simulink model "Implementation"  (Simulink 7.8)
settings: Solver=FixedStepDiscrete  StartTime=0.0  StopTime=inf  FixedStep=T  RelTol=1e-3
values from neighbouring files (symbols this model uses):
  A = [zeros(2,2),    eye(2,2) ... (first row only)    [StateFeedback_Controller_Observer_Design.m]    (also in equilibriumpositon_2_realsim.mat = [0 0 1.86000056553 -118.859256664 0 0 -4.86792536172 -131.56)
  B = [zeros(2,2) ... (first row only)    [StateFeedback_Controller_Observer_Design.m]    (also in equilibriumpositon_2_realsim.mat = [0 0 0.0946459156765 0.178753935587])
  C = [h*q2dot   h*(q1dot+q2dot) ... (first row only)    [NonLinModel.m]    (also in StateFeedback_Controller_Observer_Design.m = [1 0 0 0; equilibriumpositon_2_realsim.mat = [1  0  0  0; 0  1  0  0])
  K = place(A,B,p)    [StateFeedback_Controller_Observer_Design.m]    (also in equilibriumpositon_2_realsim.mat = [3103.64468197 1789.25362632 433.04949119 3.48374472995])
  L = transpose(place(A', C',po))    [StateFeedback_Controller_Observer_Design.m]    (also in equilibriumpositon_2_realsim.mat = [220.529108681  -24.0242041595; -32.2456951439  226.07999002)
  NewPanto = 1    [StateFeedback_Controller_Observer_Design.m]    (also in equilibriumpositon_2_realsim.mat = 0)
  q1 = x(1)    [NonLinModel.m]    (also in StateFeedback_Controller_Observer_Design.m = 1.57079632679; equilibriumpositon_2_realsim.mat = 1.57079632679)
  q2 = x(2)    [NonLinModel.m]    (also in StateFeedback_Controller_Observer_Design.m = 0; equilibriumpositon_2_realsim.mat = 3.14159265359)
  T = .001    (= 0.001)    [StateFeedback_Controller_Observer_Design.m]    (also in equilibriumpositon_2_realsim.mat)
undefined symbols (not defined in the file or in its folder): DiscIntNeverNeededParam, HIL, qc_get_step_size
libraries: quarc_library x5
settings Model: Creator=jafarm2  LastModifiedBy=jafarm2  SimulationMode=external  ExtModeTrigDuration=500000
settings SolverCC: PositivePriorityOrder=on
settings RTWCC: SystemTargetFile=quarc_win64.tlc  TemplateMakefile=quarc_default_tmf  Description=QUARC Win64 Target  ProcessScript=quarc_win64_make_rtw_hook
settings STFCustomTargetCC: TargetPreCompLibLocation=C:\PROGRA~3\QUARC\lib\2011b\win64\release  SystemTargetFile=quarc_win64.tlc
settings GRTTargetCC: TargetPreCompLibLocation=C:\PROGRA~3\QUARC\lib\2011b\win64\release  ParMdlRefBuildCompliant=off  CompOptLevelCompliant=off  ConcurrentExecutionCompliant=off  MatFileLogging=off  ExtMode=on  ExtModeMexFile=quarc_comm

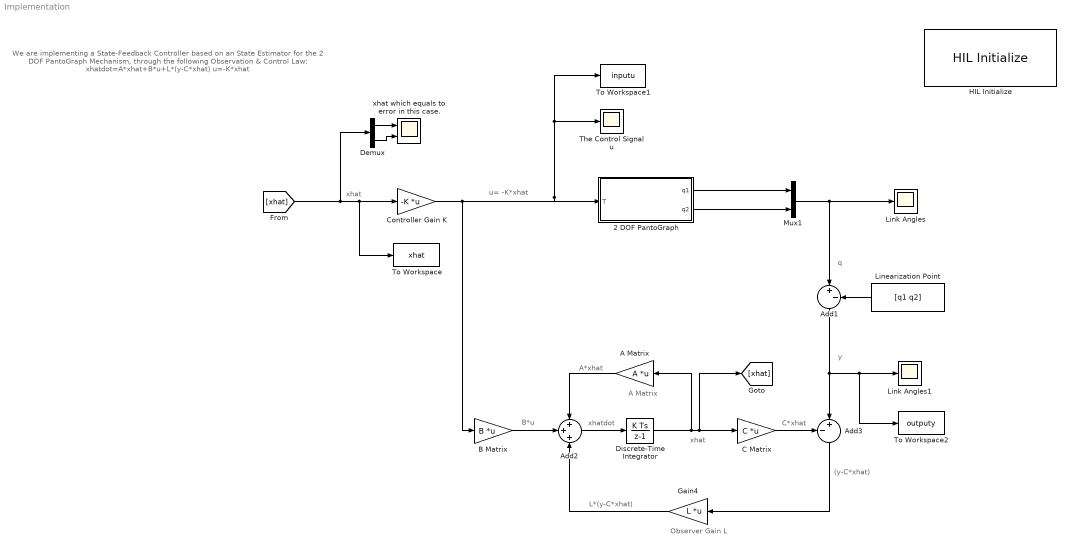
== system Implementation ==
  note: q
  note: y
  note: B*u
  note: A Matrix
  note: A*xhat
  note: xhat
  note: C*xhat
  note: (y-C*xhat)
  note: L*(y-C*xhat)
  note: Observer Gain L
  note: u= -K*xhat
  note: xhat
  note: xhatdot
  note: We are implementing a State-Feedback Controller based on an State Estimator for the 2 DOF PantoGraph Mechanism,
      | through the following Observation & Control Law:
      | xhatdot=A*xhat+B*u+L*(y-C*xhat)
      | u=-K*xhat
  2 DOF PantoGraph : Subsystem
  A Matrix : Gain  Gain=A  Multiplication=Matrix(K*u)
  Add1 : Sum  Inputs=|+-
  Add2 : Sum  Inputs=+++
  Add3 : Sum  Inputs=-+|
  B Matrix : Gain  Gain=B  Multiplication=Matrix(K*u)
  C Matrix : Gain  Gain=C  Multiplication=Matrix(K*u)
  Controller Gain K : Gain  Gain=-K  Multiplication=Matrix(K*u)
  Demux : Demux  Outputs=2
  Discrete-Time Integrator : DiscreteIntegrator  InitialCondition=[0 0 0 0]'  SampleTime=T  ICPrevOutput=DiscIntNeverNeededParam  ICPrevScaledInput=DiscIntNeverNeededParam
  Gain4 : Gain  Gain=L  Multiplication=Matrix(K*u)
  HIL Initialize : quarc_library/Data Acquisition/Generic/Configuration/HIL Initialize  object_name=HIL-2  board_type=q4  board_number=0  exclusive=off  active=on  hardware_clocks=[0:1]  clock_modes=[0 0]  initial_clock_frequencies=[]  set_clock_params_at_start=on  set_clock_params_at_switch_in=off  set_clock_frequencies_at_start=off  set_clock_frequencies_at_switch_in=off  analog_input_channels=[0:3]  analog_input_maximums=10  analog_input_minimums=-10  set_analog_input_params_at_start=off  set_analog_input_params_at_switch_in=off  analog_output_channels=[0:3]  analog_output_maximums=[10]  analog_output_minimums=[-10]  initial_analog_outputs=[0]  final_analog_outputs=[0]  watchdog_analog_outputs=0  set_analog_output_params_at_start=on  set_analog_output_params_at_switch_in=off  set_analog_outputs_at_start=on  set_analog_outputs_at_switch_in=off  set_analog_outputs_at_terminate=on  set_analog_outputs_at_switch_out=off  set_analog_outputs_on_watchdog=off  digital_input_channels=[]  digital_output_channels=[0:3]  digital_output_configuration=[]  initial_digital_outputs=[1]  final_digital_outputs=[1]  watchdog_digital_outputs=[2]  set_digital_output_params_at_start=off  set_digital_output_params_at_switch_in=off  set_digital_outputs_at_start=on  set_digital_outputs_at_switch_in=off  set_digital_outputs_at_terminate=on  set_digital_outputs_at_switch_out=off  set_digital_outputs_on_watchdog=off  encoder_channels=[0:3]  quadrature=[4]  encoder_filter_frequency=(1/60e-9)/1  initial_encoder_counts=[0]  set_encoder_params_at_start=on  set_encoder_params_at_switch_in=off  set_encoder_counts_at_start=on  set_encoder_counts_at_switch_in=off  pwm_channels=[]  pwm_modes=[0]  pwm_frequency=(1/60e-9)/1024  pwm_configuration=[]  pwm_alignment=[]  pwm_polarity=[]  pwm_leading_deadband=[]  pwm_trailing_deadband=[]  initial_pwm_outputs=[0]  final_pwm_outputs=[0]  watchdog_pwm_outputs=[]  set_pwm_params_at_start=on  set_pwm_params_at_switch_in=off  set_pwm_outputs_at_start=on  set_pwm_outputs_at_switch_in=off  set_pwm_outputs_at_terminate=on  set_pwm_outputs_at_switch_out=off  set_pwm_outputs_on_watchdog=off  other_output_channels=[]  initial_other_outputs=[]  final_other_outputs=[]  watchdog_other_outputs=[]  set_other_outputs_at_start=off  set_other_outputs_at_switch_in=off  set_other_outputs_at_terminate=off  set_other_outputs_at_switch_out=off  set_other_outputs_on_watchdog=off
  Linearization Point : Constant  Value=[q1 q2]
  Link Angles : Scope
      settings: TimeRange=30  YMin=1.5  YMax=3.2
  Link Angles1 : Scope
      settings: TimeRange=60  YMin=0  YMax=0.017  SaveName=ScopeData4
  Mux1 : Mux  Inputs=2
  The Control Signal u : Scope
      settings: TimeRange=30  YMin=-300  YMax=300  SaveName=ScopeData3
  To Workspace : ToWorkspace  VariableName=xhat  SampleTime=-1  SaveFormat=Structure
  To Workspace1 : ToWorkspace  VariableName=inputu  SampleTime=-1  SaveFormat=Structure
  To Workspace2 : ToWorkspace  VariableName=outputy  SampleTime=-1  SaveFormat=Structure
  xhat which equals to error in this case. : Scope  NumInputPorts=2
      settings: YMin=-0.003~-0.15  YMax=0.0045~0.15
  wires:
  Controller Gain K/1 -> B Matrix/1, The Control Signal u/1, To Workspace1/1, 2 DOF PantoGraph/1(T)
  Mux1/1 -> Link Angles/1, Add1/1
  2 DOF PantoGraph/1(q1) -> Mux1/1
  2 DOF PantoGraph/2(q2) -> Mux1/2
  Add2/1 -> Discrete-Time Integrator/1
  C Matrix/1 -> Add3/1
  Add3/1 -> Gain4/1
  Discrete-Time Integrator/1 -> A Matrix/1, C Matrix/1, [xhat]
  B Matrix/1 -> Add2/2
  A Matrix/1 -> Add2/1
  Add1/1 -> Add3/2, Link Angles1/1, To Workspace2/1
  Linearization Point/1 -> Add1/2
  Gain4/1 -> Add2/3
  [xhat] -> Demux/1, To Workspace/1, Controller Gain K/1
  Demux/1 -> xhat which equals to error in this case./1
  Demux/2 -> xhat which equals to error in this case./2

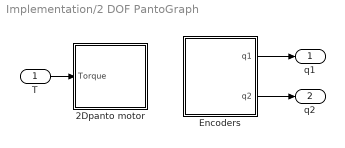
== system Implementation/2 DOF PantoGraph ==
  T : Inport
  2Dpanto motor : Subsystem
  Encoders : Subsystem
  q1 : Outport
  q2 : Outport  Port=2
  wires:
  T/1 -> 2Dpanto motor/1(Torque)
  Encoders/1(q1) -> q1/1
  Encoders/2(q2) -> q2/1

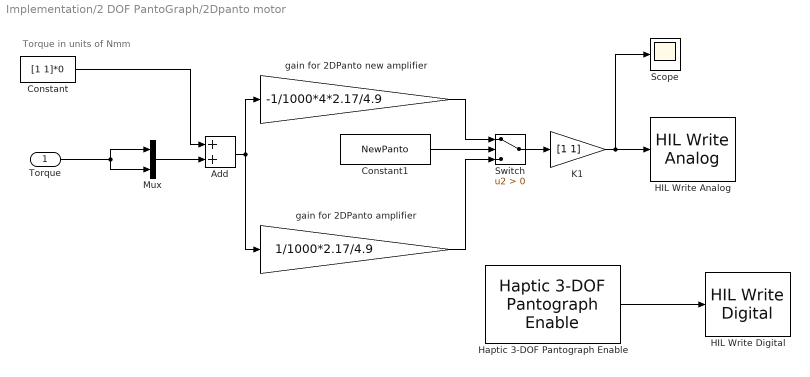
== system Implementation/2 DOF PantoGraph/2Dpanto motor ==
  note: Torque in units of Nmm
  Torque : Inport
  Add : Sum
  Constant : Constant  Value=[1 1]*0
  Constant1 : Constant  Value=NewPanto
  HIL Write Analog : quarc_library/Data Acquisition/Generic/Immediate I//O/HIL Write Analog  object_name=HIL-2  channels=[0:1]  sample_time=-1  active=off  vector_input=on
  HIL Write Digital : quarc_library/Data Acquisition/Generic/Immediate I//O/HIL Write Digital  object_name=HIL-2  channels=0:3  sample_time=-1  active=off  vector_input=on
  Haptic 3-DOF Pantograph Enable : quarc_library/Devices/Quanser/Haptics/Pantographs/Haptic 3-DOF Planar Pantograph/Interfacing/Haptic 3-DOF Pantograph Enable
  K1 : Gain  Gain=[1 1]
  Mux : Mux  Inputs=2
  Scope : Scope
      settings: SaveName=ScopeData2
  Switch : Switch  Criteria=u2 > Threshold
  gain for 2DPanto amplifier : Gain  Gain=1/1000*2.17/4.9
  gain for 2DPanto new amplifier : Gain  Gain=-1/1000*4*2.17/4.9
  wires:
  Constant/1 -> Add/1
  K1/1 -> HIL Write Analog/1, Scope/1
  Add/1 -> gain for 2DPanto amplifier/1, gain for 2DPanto new amplifier/1
  Switch/1 -> K1/1
  gain for 2DPanto new amplifier/1 -> Switch/1
  gain for 2DPanto amplifier/1 -> Switch/3
  Constant1/1 -> Switch/2
  Torque/1 -> Mux/1, Mux/2
  Haptic 3-DOF Pantograph Enable/1 -> HIL Write Digital/1
  Mux/1 -> Add/2

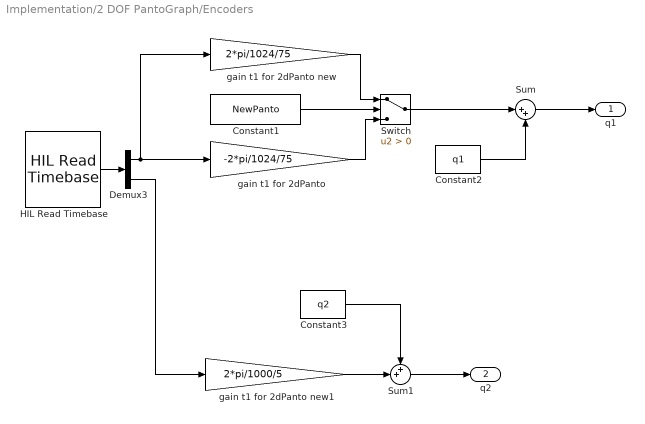
== system Implementation/2 DOF PantoGraph/Encoders ==
  Constant1 : Constant  Value=NewPanto
  Constant2 : Constant  Value=q1
  Constant3 : Constant  Value=q2
  Demux3 : Demux  Outputs=3
  HIL Read Timebase : quarc_library/Data Acquisition/Generic/Timebases/HIL Read Timebase  object_name=HIL-2  clock=0  analog_channels=[]  encoder_channels=[0:2]  digital_channels=[]  other_channels=[]  samples_in_buffer=max(ceil(1/qc_get_step_size), 1)  active=on  vector_output=on  data_type_mode=Inherit via back propagation  encoder_data_type=double  digital_data_type=boolean
  Sum : Sum  Inputs=|++
  Sum1 : Sum  Inputs=++|
  Switch : Switch  Criteria=u2 > Threshold
  gain t1 for 2dPanto : Gain  Gain=-2*pi/1024/75
  gain t1 for 2dPanto new : Gain  Gain=2*pi/1024/75
  gain t1 for 2dPanto new1 : Gain  Gain=2*pi/1000/5
  q1 : Outport
  q2 : Outport  Port=2
  wires:
  HIL Read Timebase/1 -> Demux3/1
  Demux3/1 -> gain t1 for 2dPanto/1, gain t1 for 2dPanto new/1
  gain t1 for 2dPanto new/1 -> Switch/1
  gain t1 for 2dPanto/1 -> Switch/3
  Constant1/1 -> Switch/2
  Demux3/3 -> gain t1 for 2dPanto new1/1
  Switch/1 -> Sum/1
  Sum/1 -> q1/1
  Constant2/1 -> Sum/2
  Constant3/1 -> Sum1/1
  gain t1 for 2dPanto new1/1 -> Sum1/2
  Sum1/1 -> q2/1
